simulink model "svlvvpr1_schema_SVLVV"  (R2020a)
settings: Solver=VariableStepAuto  StartTime=0.0  StopTime=10.0  RelTol=1e-3
values from neighbouring files (symbols this model uses):
  w = ws(i)    [svlvv1_skript.m]
settings Model: Creator=dot  LastModifiedBy=dot

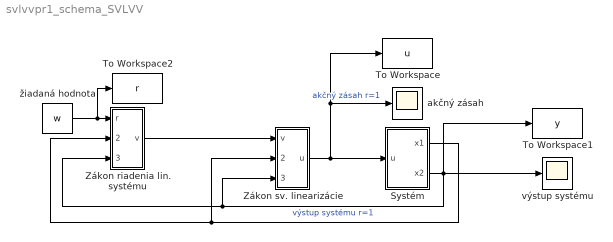
== system svlvvpr1_schema_SVLVV ==
  Systém : Subsystem
  To Workspace : ToWorkspace  VariableName=u  SaveFormat=Timeseries  SampleTime=-1
  To Workspace1 : ToWorkspace  VariableName=y  SaveFormat=Timeseries  SampleTime=-1
  To Workspace2 : ToWorkspace  VariableName=r  SaveFormat=Timeseries  SampleTime=-1
  Zákon riadenia lin. systému : Subsystem
  Zákon sv. linearizácie : Subsystem
  akčný zásah : Scope
  výstup systému : Scope
  žiadaná hodnota : Constant  Value=w
  wires:
  Systém/2(x2) -> To Workspace1/1, výstup systému/1, Zákon sv. linearizácie/3(x2), Zákon riadenia lin. systému/3(x2)  "výstup systému r=1"
  Systém/1(x1) -> Zákon sv. linearizácie/2(x1), Zákon riadenia lin. systému/2(x1)
  Zákon sv. linearizácie/1(u) -> To Workspace/1, akčný zásah/1, Systém/1(u)  "akčný zásah r=1"
  žiadaná hodnota/1 -> To Workspace2/1, Zákon riadenia lin. systému/1(r)
  Zákon riadenia lin. systému/1(v) -> Zákon sv. linearizácie/1(v)

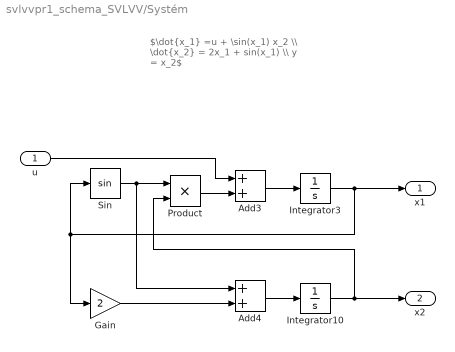
== system svlvvpr1_schema_SVLVV/Systém ==
  note: $\dot{x_1} =u + \sin(x_1) x_2 \\ \dot{x_2} = 2x_1 + sin(x_1) \\ y = x_2$
  u : Inport
  Add3 : Sum
  Add4 : Sum
  Gain : Gain  Gain=2
  Integrator10 : Integrator
  Integrator3 : Integrator
  Product : Product
  Sin : Trigonometry
  x1 : Outport
  x2 : Outport  Port=2
  wires:
  Add4/1 -> Integrator10/1
  Gain/1 -> Add4/2
  u/1 -> Add3/1
  Add3/1 -> Integrator3/1
  Integrator3/1 -> Sin/1, Gain/1, x1/1
  Product/1 -> Add3/2
  Integrator10/1 -> Product/2, x2/1
  Sin/1 -> Product/1, Add4/1

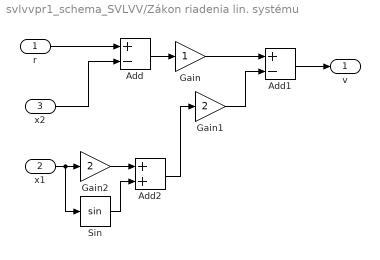
== system svlvvpr1_schema_SVLVV/Zákon riadenia lin. systému ==
  r : Inport
  x1 : Inport  Port=2
  x2 : Inport  Port=3
  Add : Sum  Inputs=+-
  Add1 : Sum  Inputs=+-
  Add2 : Sum
  Gain : Gain
  Gain1 : Gain  Gain=2
  Gain2 : Gain  Gain=2
  Sin : Trigonometry
  v : Outport
  wires:
  r/1 -> Add/1
  x1/1 -> Sin/1, Gain2/1
  Add/1 -> Gain/1
  Gain/1 -> Add1/1
  Add1/1 -> v/1
  Gain1/1 -> Add1/2
  Gain2/1 -> Add2/1
  Sin/1 -> Add2/2
  Add2/1 -> Gain1/1
  x2/1 -> Add/2

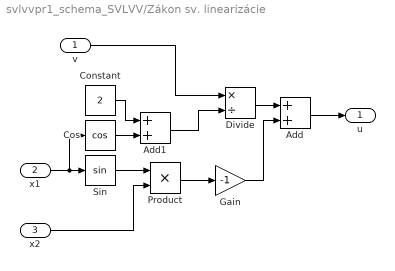
== system svlvvpr1_schema_SVLVV/Zákon sv. linearizácie ==
  v : Inport
  x1 : Inport  Port=2
  x2 : Inport  Port=3
  Add : Sum
  Add1 : Sum
  Constant : Constant  Value=2
  Cos : Trigonometry  Operator=cos
  Divide : Product  Inputs=*/
  Gain : Gain  Gain=-1
  Product : Product
  Sin : Trigonometry
  u : Outport
  wires:
  x1/1 -> Cos/1, Sin/1
  Sin/1 -> Product/1
  x2/1 -> Product/2
  Product/1 -> Gain/1
  Add/1 -> u/1
  Gain/1 -> Add/2
  Cos/1 -> Add1/2
  Constant/1 -> Add1/1
  Divide/1 -> Add/1
  v/1 -> Divide/1
  Add1/1 -> Divide/2
